simulink model "FYI_Twin_CyberResilient"  (R2025b)
settings: Solver=VariableStepAuto  StartTime=0.0  StopTime=TF  FixedStep=1/120  RelTol=1e-5
PreLoadFcn:
  | [aircraft, state] = astDehavillandBeaver();
  | thrustX = getCoefficient(aircraft,"CX","Propeller",Component="Propeller");
model workspace (MATLAB code in the model file + MAT data in the model file):
  ActuatorCmds = [0.0013469; -0.14185; -0.03733]
  AileronCmd = 0.0013469
  ElevatorCmd = -0.14185
  RudderCmd = -0.03733
  TF = 60
  ThrottleCmd = 0.5
  U0 = 33.0529
  V0 = 0.093272
  W0 = 10.1004
  Xe0 = -2.8165e-12
  Ye0 = 4.3033e-12
  Ze0 = -2202
  aircraft : Aero.FixedWing (value not decoded)
  altitude0 = 2202
  attack_enable = 1
  attack_mode = 3
  blend_rate = 0.05
  inputs0 : object (value not decoded)
  lat0 = 0.843936506509
  lat0_deg = 48.354
  lon0 = 0.205746393542
  lon0_deg = 11.7884
  p0 = 3.0707e-20
  phi0 = 0.0092342
  psi0 = 0
  q0 = 5.1124e-22
  r0 = -8.6217e-20
  required_count = 5
  state : astDehavillandBeaverState (value not decoded)
  states : object (value not decoded)
  states0 : object (value not decoded)
  theta0 = 0.29658
  thrustX : Simulink.LookupTable (value not decoded)
  u_twin = [0.0013469; -0.14185; -0.03733; 0.5; 0.5]
  x0 = [0.0092342; 0.29658; 0; 3.0707e-20; 5.1124e-22; -8.6217e-20; 33.0529; 0.093272; 10.1004; -2.8165e-12; 4.3033e-12; -2202]
  x0_beaver = [0.0092342; 0.29658; 0; 3.0707e-20; 5.1124e-22; -8.6217e-20; 33.0529; 0.093272; 10.1004; -2.8165e-12; 4.3033e-12; -8202]
  x0_unified = [33.0529; 0.093272; 10.1004; 0.0092342; 0.29658; 0; 3.0707e-20; 5.1124e-22; -8.6217e-20; 0.205746393542; 0.843936506509; 2202]
  other statements: initialize6DOFSkyHogg;
symbols that are objects in the model workspace (value not decoded): aircraft, state
undefined symbols (not defined in the file or in its folder): F, Light, MIL
libraries: aerolibasang x6, aerolibobsolete x2, aerolibadyn x2, aerolibatmos2 x2, aerolibwind2 x2, sharedtransform x2, aerolibfltsims x2
(part 2 of 2)

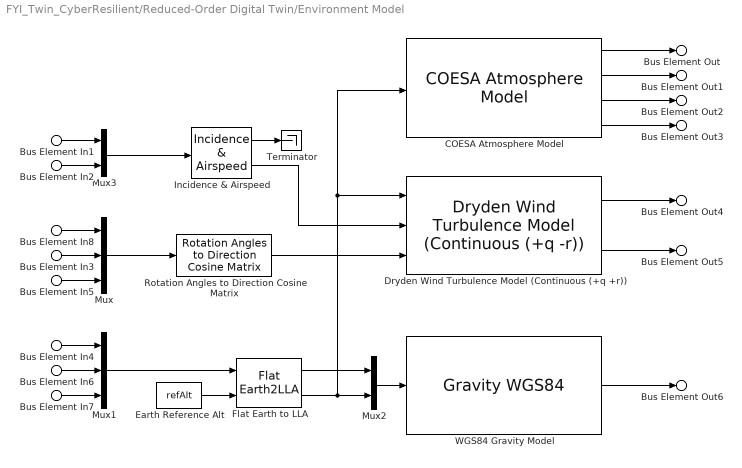
== system FYI_Twin_CyberResilient/Reduced-Order Digital Twin/Environment Model ==
  Bus Element In1 : Inport  PortName=States  Element=u
  Bus Element In2 : Inport  PortName=States  Element=w
  Bus Element In3 : Inport  PortName=States  Element=theta
  Bus Element In4 : Inport  PortName=States  Element=Xe
  Bus Element In7 : Inport  PortName=States  Element=Ze
  Bus Element In8 : Inport  PortName=States  Element=phi
  Bus Element In5 : Inport  PortName=States  Element=psi
  Bus Element In6 : Inport  PortName=States  Element=Ye
  COESA Atmosphere Model : aerolibatmos2/COESA Atmosphere Model  units=Metric (MKS)  spec=1976 COESA-extended U.S. Standard Atmosphere  model=Profile  profile_var=High temperature  profile_percent=1%  profile_alt=5 km (16404 ft)  envelope_var=High temperature  envelope_percent=1%  action=Warning
  Dryden Wind Turbulence Model (Continuous (+q +r)) : aerolibwind2/Dryden Wind Turbulence Model  (Continuous (+q -r))  units=Metric (MKS)  spec=MIL-F-8785C  model=Continuous Dryden (+q -r)  W20=W20  Wdeg=Wdeg  TurbProb=10^-2 - Light  L_high=L_high  Wingspan=Wingspan  ts=ts  Seed=Seed  T_on=off
  Earth Reference Alt : Constant  Value=refAlt
  Flat Earth to LLA : FlatEarth2LLA  R=6378137  LL0=[0 0]
  Incidence & Airspeed : aerolibasang/Incidence  & Airspeed
  Mux : Mux  Inputs=3
  Mux1 : Mux  Inputs=3
  Mux2 : Mux  Inputs=2
  Mux3 : Mux  Inputs=2
  Rotation Angles to Direction Cosine Matrix : sharedtransform/Rotation Angles to Direction Cosine Matrix  rotationOrder=ZYX  aMode=aMode
  Terminator : Terminator
  "WGS84 Gravity Model  " : GravityWGS84
  Bus Element Out : Outport  VectorParamsAs1DForOutWhenUnconnected=off  PortName=Env  Element=To
  Bus Element Out1 : Outport  VectorParamsAs1DForOutWhenUnconnected=off  PortName=Env  Element=a
  Bus Element Out2 : Outport  VectorParamsAs1DForOutWhenUnconnected=off  PortName=Env  Element=Po
  Bus Element Out3 : Outport  VectorParamsAs1DForOutWhenUnconnected=off  PortName=Env  Element=AirDensity
  Bus Element Out4 : Outport  VectorParamsAs1DForOutWhenUnconnected=off  PortName=Env  Element=WindVelocity
  Bus Element Out5 : Outport  VectorParamsAs1DForOutWhenUnconnected=off  PortName=Env  Element=WindAngularRates
  Bus Element Out6 : Outport  VectorParamsAs1DForOutWhenUnconnected=off  PortName=Env  Element=g
  wires:
  Dryden Wind Turbulence Model (Continuous (+q +r))/1 -> Bus Element Out4/1
  Dryden Wind Turbulence Model (Continuous (+q +r))/2 -> Bus Element Out5/1
  Mux2/1 -> "WGS84 Gravity Model  "/1
  Bus Element In4/1 -> Mux1/1
  Bus Element In7/1 -> Mux1/3
  Bus Element In6/1 -> Mux1/2
  Bus Element In5/1 -> Mux/3
  Bus Element In8/1 -> Mux/1
  Bus Element In2/1 -> Mux3/2
  Bus Element In1/1 -> Mux3/1
  "WGS84 Gravity Model  "/1 -> Bus Element Out6/1
  COESA Atmosphere Model/2 -> Bus Element Out1/1
  COESA Atmosphere Model/1 -> Bus Element Out/1
  COESA Atmosphere Model/4 -> Bus Element Out3/1
  COESA Atmosphere Model/3 -> Bus Element Out2/1
  Flat Earth to LLA/1 -> Mux2/1
  Earth Reference Alt/1 -> Flat Earth to LLA/2
  Incidence & Airspeed/2 -> Dryden Wind Turbulence Model (Continuous (+q +r))/2
  Flat Earth to LLA/2 -> Mux2/2, COESA Atmosphere Model/1, Dryden Wind Turbulence Model (Continuous (+q +r))/1
  Mux3/1 -> Incidence & Airspeed/1
  Incidence & Airspeed/1 -> Terminator/1
  Mux/1 -> Rotation Angles to Direction Cosine Matrix/1
  Bus Element In3/1 -> Mux/2
  Rotation Angles to Direction Cosine Matrix/1 -> Dryden Wind Turbulence Model (Continuous (+q +r))/3
  Mux1/1 -> Flat Earth to LLA/1

== system FYI_Twin_CyberResilient/Reduced-Order Digital Twin/Propulsion ==
  cmd : Inport
  Mux : Mux  Inputs=[1 2]
  ThrustX : Lookup_n-D  NumberOfTableDimensions=1  DataSpecification=Lookup table object  LookupTableObject=thrustX  BreakpointsForDimension1="getCoefficient(aircraft,\"CX\",\"Propeller\",Component=\"Propeller\").Breakpoints(1).Value"  IndexSearchMethod=Linear search  BeginIndexSearchUsingPreviousIndexResult=on  Table="getCoefficient(aircraft,\"CX\",\"Propeller\",Component=\"Propeller\").Table.Value"  ExtrapMethod=Clip
  ThrustYZ : Constant  Value=[0 0]'  SampleTime=-1
  Thrust_M1 : Constant  Value=[0 0 0]'  SampleTime=-1
  F : Outport  Unit=N  VectorParamsAs1DForOutWhenUnconnected=off
  M : Outport  Port=2  Unit=N*m  VectorParamsAs1DForOutWhenUnconnected=off
  wires:
  Thrust_M1/1 -> M/1
  ThrustX/1 -> Mux/1
  ThrustYZ/1 -> Mux/2
  Mux/1 -> F/1
  cmd/1 -> ThrustX/1

== system FYI_Twin_CyberResilient/True Aircraft States Adapter/Geodetic Coordinates ==
  VN : Inport
  VE : Inport  Port=2
  VD : Inport  Port=3
  Gain : Gain  Gain=-1
  Integrator : Integrator  InitialCondition=150
  Integrator1 : Integrator  InitialCondition=0.22181
  Integrator2 : Integrator  InitialCondition=1.356068
  LATITUDE : MATLAB Function  TreatAsAtomicUnit=on
  LONGITUDE : MATLAB Function  TreatAsAtomicUnit=on
  M and N : Subsystem
  gamma(Longitude) : Outport
  phi(Latitude) : Outport  Port=2
  h : Outport  Port=3
  wires:
  VD/1 -> Gain/1  "VD"
  Gain/1 -> Integrator/1  "h_dot"
  Integrator/1 -> LATITUDE/3(h), LONGITUDE/3(h), h/1  "h"
  M and N/1(M) -> LATITUDE/2(M)
  M and N/2(N) -> LONGITUDE/2(N)
  LATITUDE/1(phi_dot) -> Integrator1/1  "phi_dot"
  Integrator1/1 -> LONGITUDE/4(phi), M and N/1(phi), phi(Latitude)/1  "phi"
  VE/1 -> LONGITUDE/1(VE)  "VE"
  VN/1 -> LATITUDE/1(VN)  "VN"
  LONGITUDE/1(gamma_dot) -> Integrator2/1  "gamma_dot"
  Integrator2/1 -> gamma(Longitude)/1  "gamma"

== system FYI_Twin_CyberResilient/True Aircraft States Adapter/Navigational BLOCK ==
  U : Inport
  V : Inport  Port=2
  W : Inport  Port=3
  Phi : Inport  Port=4
  Theta : Inport  Port=5
  Psi : Inport  Port=6
  Math Function : Math  Operator=transpose
  Matrix Multiply : Product  Multiplication=Matrix(*)
  Mux2 : Mux  Inputs=3
  Navigational Equation : Subsystem
  V_v : Outport
  wires:
  V/1 -> Mux2/2
  Psi/1 -> Navigational Equation/3(phi)
  W/1 -> Mux2/3
  Navigational Equation/1(C_B/V) -> Math Function/1
  Matrix Multiply/1 -> V_v/1
  Theta/1 -> Navigational Equation/2(theat)
  U/1 -> Mux2/1
  Phi/1 -> Navigational Equation/1(psi)
  Math Function/1 -> Matrix Multiply/1
  Mux2/1 -> Matrix Multiply/2

== system FYI_Twin_CyberResilient/Twin_States_Adapter/Geodetic Coordinates ==
  VN : Inport
  VE : Inport  Port=2
  VD : Inport  Port=3
  Gain : Gain  Gain=-1
  Integrator : Integrator  InitialCondition=150
  Integrator1 : Integrator  InitialCondition=0.22181
  Integrator2 : Integrator  InitialCondition=1.356068
  LATITUDE : MATLAB Function  TreatAsAtomicUnit=on
  LONGITUDE : MATLAB Function  TreatAsAtomicUnit=on
  M and N : Subsystem
  gamma(Longitude) : Outport
  phi(Latitude) : Outport  Port=2
  h : Outport  Port=3
  wires:
  VD/1 -> Gain/1  "VD"
  Gain/1 -> Integrator/1  "h_dot"
  Integrator/1 -> LATITUDE/3(h), LONGITUDE/3(h), h/1  "h"
  M and N/1(M) -> LATITUDE/2(M)
  M and N/2(N) -> LONGITUDE/2(N)
  LATITUDE/1(phi_dot) -> Integrator1/1  "phi_dot"
  Integrator1/1 -> LONGITUDE/4(phi), M and N/1(phi), phi(Latitude)/1  "phi"
  VE/1 -> LONGITUDE/1(VE)  "VE"
  VN/1 -> LATITUDE/1(VN)  "VN"
  LONGITUDE/1(gamma_dot) -> Integrator2/1  "gamma_dot"
  Integrator2/1 -> gamma(Longitude)/1  "gamma"

== system FYI_Twin_CyberResilient/Twin_States_Adapter/Navigational BLOCK ==
  U : Inport
  V : Inport  Port=2
  W : Inport  Port=3
  Phi : Inport  Port=4
  Theta : Inport  Port=5
  Psi : Inport  Port=6
  Math Function : Math  Operator=transpose
  Matrix Multiply : Product  Multiplication=Matrix(*)
  Mux2 : Mux  Inputs=3
  Navigational Equation : Subsystem
  V_v : Outport
  wires:
  V/1 -> Mux2/2
  Psi/1 -> Navigational Equation/3(phi)
  W/1 -> Mux2/3
  Navigational Equation/1(C_B/V) -> Math Function/1
  Matrix Multiply/1 -> V_v/1
  Theta/1 -> Navigational Equation/2(theat)
  U/1 -> Mux2/1
  Phi/1 -> Navigational Equation/1(psi)
  Math Function/1 -> Matrix Multiply/1
  Mux2/1 -> Matrix Multiply/2

== system FYI_Twin_CyberResilient/6-DoF Aircraft Plant/Aerodynamic Model/Actuator Aerodynamic Coefficients ==
  Bus Element In13 : Inport  PortName=ActuatorCmds  Element=Elevator
  Bus Element In1 : Inport  PortName=ActuatorCmds  Element=Aileron
  Bus Element In2 : Inport  PortName=ActuatorCmds  Element=Rudder
  Alpha : Inport  Port=2
  Beta2 : Inport  Port=3
  Aileron : Subsystem
  Constant : Constant  Value=0
  Elevator : Subsystem
  Flap : Subsystem
  Rudder : Subsystem
  Sum : Sum  Inputs=4  InputSameDT=on  SaturateOnIntegerOverflow=on  OutDataTypeStr=Inherit: Same as first input
  Coeff : Outport  InitialOutput=0  VectorParamsAs1DForOutWhenUnconnected=off
  wires:
  Constant/1 -> Flap/1(Actuator)
  Bus Element In2/1 -> Rudder/1(Actuator)
  Bus Element In1/1 -> Aileron/1(Actuator)
  Bus Element In13/1 -> Elevator/1(Actuator)
  Beta2/1 -> Elevator/2(Beta2)
  Flap/1(delCoeff) -> Sum/4
  Alpha/1 -> Flap/2(Alpha), Rudder/2(Alpha), Aileron/2(Alpha)
  Rudder/1(delCoeff) -> Sum/3
  Aileron/1(delCoeff) -> Sum/2
  Elevator/1(delCoeff) -> Sum/1
  Sum/1 -> Coeff/1

== system FYI_Twin_CyberResilient/6-DoF Aircraft Plant/Aerodynamic Model/Aerodynamic Coefficients ==
  Alpha : Inport
  Alpha2 : Inport  Port=2
  Alpha3 : Inport  Port=3
  Beta : Inport  Port=4
  Beta2 : Inport  Port=5
  Beta3 : Inport  Port=6
  V : Inport  Port=7
  pqr : Inport  Port=8  Unit=m/s
  Body Rate Damping : Subsystem
  Datum Coefficients : Subsystem
  Sum : Sum  Inputs=|++
  Coeff : Outport  VectorParamsAs1DForOutWhenUnconnected=off
  wires:
  pqr/1 -> Body Rate Damping/2(pqr)
  Sum/1 -> Coeff/1
  V/1 -> Body Rate Damping/1(V)
  Body Rate Damping/1(Coeff) -> Sum/2
  Datum Coefficients/1(Coeff) -> Sum/1
  Beta/1 -> Datum Coefficients/4(Beta)
  Alpha/1 -> Datum Coefficients/1(Alpha)
  Alpha2/1 -> Datum Coefficients/2(Alpha2)
  Alpha3/1 -> Datum Coefficients/3(Alpha3)
  Beta2/1 -> Datum Coefficients/5(Beta2)
  Beta3/1 -> Datum Coefficients/6(Beta3)

== system FYI_Twin_CyberResilient/6-DoF Aircraft Plant/Aerodynamic Model/Subsystem ==
  Vb : Inport
  "Incidence, Sideslip, & Airspeed" : aerolibasang/Incidence, Sideslip, & Airspeed
  Product{,1..3} (4 alike) : Product
  Alpha : Outport
  Alpha2 : Outport  Port=2
  Alpha3 : Outport  Port=3
  Beta : Outport  Port=4
  Beta2 : Outport  Port=5
  Beta3 : Outport  Port=6
  V : Outport  Port=7
  wires:
  Product/1 -> Product1/1, Alpha2/1
  "Incidence, Sideslip, & Airspeed"/1 -> Product/1, Alpha/1, Product/2, Product1/2
  "Incidence, Sideslip, & Airspeed"/3 -> V/1
  Vb/1 -> "Incidence, Sideslip, & Airspeed"/1
  Product1/1 -> Alpha3/1
  Product2/1 -> Product3/1, Beta2/1
  Product3/1 -> Beta3/1
  "Incidence, Sideslip, & Airspeed"/2 -> Product3/2, Product2/2, Product2/1, Beta/1

== system FYI_Twin_CyberResilient/6-DoF Aircraft Plant/Aerodynamic Model/ToBus ==
  I : Inport
  Bus Creator3 : BusCreator  Inputs=3
  Demux : Demux  Outputs=3
  O : Outport  VectorParamsAs1DForOutWhenUnconnected=off
  wires:
  I/1 -> Demux/1
  Demux/2 -> Bus Creator3/2  "q_wind"
  Bus Creator3/1 -> O/1
  Demux/3 -> Bus Creator3/3  "r_wind"
  Demux/1 -> Bus Creator3/1  "p_wind"

== system FYI_Twin_CyberResilient/Reduced-Order Digital Twin/Aerodynamic Model/Actuator Aerodynamic Coefficients ==
  Bus Element In13 : Inport  PortName=ActuatorCmds  Element=Elevator
  Bus Element In1 : Inport  PortName=ActuatorCmds  Element=Aileron
  Bus Element In2 : Inport  PortName=ActuatorCmds  Element=Rudder
  Alpha : Inport  Port=2
  Beta2 : Inport  Port=3
  Aileron : Subsystem
  Constant : Constant  Value=0
  Elevator : Subsystem
  Flap : Subsystem
  Rudder : Subsystem
  Sum : Sum  Inputs=4  InputSameDT=on  SaturateOnIntegerOverflow=on  OutDataTypeStr=Inherit: Same as first input
  Coeff : Outport  InitialOutput=0  VectorParamsAs1DForOutWhenUnconnected=off
  wires:
  Constant/1 -> Flap/1(Actuator)
  Bus Element In2/1 -> Rudder/1(Actuator)
  Bus Element In1/1 -> Aileron/1(Actuator)
  Bus Element In13/1 -> Elevator/1(Actuator)
  Beta2/1 -> Elevator/2(Beta2)
  Flap/1(delCoeff) -> Sum/4
  Alpha/1 -> Flap/2(Alpha), Rudder/2(Alpha), Aileron/2(Alpha)
  Rudder/1(delCoeff) -> Sum/3
  Aileron/1(delCoeff) -> Sum/2
  Elevator/1(delCoeff) -> Sum/1
  Sum/1 -> Coeff/1

== system FYI_Twin_CyberResilient/Reduced-Order Digital Twin/Aerodynamic Model/Aerodynamic Coefficients ==
  Alpha : Inport
  Alpha2 : Inport  Port=2
  Alpha3 : Inport  Port=3
  Beta : Inport  Port=4
  Beta2 : Inport  Port=5
  Beta3 : Inport  Port=6
  V : Inport  Port=7
  pqr : Inport  Port=8  Unit=m/s
  Body Rate Damping : Subsystem
  Datum Coefficients : Subsystem
  Sum : Sum  Inputs=|++
  Coeff : Outport  VectorParamsAs1DForOutWhenUnconnected=off
  wires:
  pqr/1 -> Body Rate Damping/2(pqr)
  Sum/1 -> Coeff/1
  V/1 -> Body Rate Damping/1(V)
  Body Rate Damping/1(Coeff) -> Sum/2
  Datum Coefficients/1(Coeff) -> Sum/1
  Beta/1 -> Datum Coefficients/4(Beta)
  Alpha/1 -> Datum Coefficients/1(Alpha)
  Alpha2/1 -> Datum Coefficients/2(Alpha2)
  Alpha3/1 -> Datum Coefficients/3(Alpha3)
  Beta2/1 -> Datum Coefficients/5(Beta2)
  Beta3/1 -> Datum Coefficients/6(Beta3)

== system FYI_Twin_CyberResilient/Reduced-Order Digital Twin/Aerodynamic Model/Subsystem ==
  Vb : Inport
  "Incidence, Sideslip, & Airspeed" : aerolibasang/Incidence, Sideslip, & Airspeed
  Product{,1..3} (4 alike) : Product
  Alpha : Outport
  Alpha2 : Outport  Port=2
  Alpha3 : Outport  Port=3
  Beta : Outport  Port=4
  Beta2 : Outport  Port=5
  Beta3 : Outport  Port=6
  V : Outport  Port=7
  wires:
  Product/1 -> Product1/1, Alpha2/1
  "Incidence, Sideslip, & Airspeed"/1 -> Product/1, Alpha/1, Product/2, Product1/2
  "Incidence, Sideslip, & Airspeed"/3 -> V/1
  Vb/1 -> "Incidence, Sideslip, & Airspeed"/1
  Product1/1 -> Alpha3/1
  Product2/1 -> Product3/1, Beta2/1
  Product3/1 -> Beta3/1
  "Incidence, Sideslip, & Airspeed"/2 -> Product3/2, Product2/2, Product2/1, Beta/1

== system FYI_Twin_CyberResilient/Reduced-Order Digital Twin/Aerodynamic Model/ToBus ==
  I : Inport
  Bus Creator3 : BusCreator  Inputs=3
  Demux : Demux  Outputs=3
  O : Outport  VectorParamsAs1DForOutWhenUnconnected=off
  wires:
  I/1 -> Demux/1
  Demux/2 -> Bus Creator3/2  "q_wind"
  Bus Creator3/1 -> O/1
  Demux/3 -> Bus Creator3/3  "r_wind"
  Demux/1 -> Bus Creator3/1  "p_wind"

== system FYI_Twin_CyberResilient/True Aircraft States Adapter/Geodetic Coordinates/M and N ==
  phi : Inport
  Constant : Constant  Value=0.081819190842622
  M and N : MATLAB Function  TreatAsAtomicUnit=on
  a : Constant  Value=6378137
  M : Outport
  N : Outport  Port=2
  wires:
  Constant/1 -> M and N/2(e)
  phi/1 -> M and N/3(phi)
  M and N/1(M) -> M/1
  a/1 -> M and N/1(a)
  M and N/2(N) -> N/1

== system FYI_Twin_CyberResilient/True Aircraft States Adapter/Navigational BLOCK/Navigational Equation ==
  psi : Inport
  theat : Inport  Port=2
  phi : Inport  Port=3
  Matrix Multiply : Product  Inputs=3  Multiplication=Matrix(*)
  Roationa Matrix from 2 to body : MATLAB Function  TreatAsAtomicUnit=on
  Roational Matrix from 1 to 2 : MATLAB Function  TreatAsAtomicUnit=on
  Rotaional Matrix from V to 1 : MATLAB Function  TreatAsAtomicUnit=on
  C_B/V : Outport
  wires:
  psi/1 -> Rotaional Matrix from V to 1/1(psi)
  theat/1 -> Roational Matrix from 1 to 2/1(theta)
  phi/1 -> Roationa Matrix from 2 to body/1(phi)
  Roationa Matrix from 2 to body/1(C_b_2) -> Matrix Multiply/1
  Roational Matrix from 1 to 2/1(C_2_1) -> Matrix Multiply/2
  Rotaional Matrix from V to 1/1(C_1_V) -> Matrix Multiply/3
  Matrix Multiply/1 -> C_B/V/1

== system FYI_Twin_CyberResilient/Twin_States_Adapter/Geodetic Coordinates/M and N ==
  phi : Inport
  Constant : Constant  Value=0.081819190842622
  M and N : MATLAB Function  TreatAsAtomicUnit=on
  a : Constant  Value=6378137
  M : Outport
  N : Outport  Port=2
  wires:
  Constant/1 -> M and N/2(e)
  phi/1 -> M and N/3(phi)
  M and N/1(M) -> M/1
  a/1 -> M and N/1(a)
  M and N/2(N) -> N/1

== system FYI_Twin_CyberResilient/Twin_States_Adapter/Navigational BLOCK/Navigational Equation ==
  psi : Inport
  theat : Inport  Port=2
  phi : Inport  Port=3
  Matrix Multiply : Product  Inputs=3  Multiplication=Matrix(*)
  Roationa Matrix from 2 to body : MATLAB Function  TreatAsAtomicUnit=on
  Roational Matrix from 1 to 2 : MATLAB Function  TreatAsAtomicUnit=on
  Rotaional Matrix from V to 1 : MATLAB Function  TreatAsAtomicUnit=on
  C_B/V : Outport
  wires:
  psi/1 -> Rotaional Matrix from V to 1/1(psi)
  theat/1 -> Roational Matrix from 1 to 2/1(theta)
  phi/1 -> Roationa Matrix from 2 to body/1(phi)
  Roationa Matrix from 2 to body/1(C_b_2) -> Matrix Multiply/1
  Roational Matrix from 1 to 2/1(C_2_1) -> Matrix Multiply/2
  Rotaional Matrix from V to 1/1(C_1_V) -> Matrix Multiply/3
  Matrix Multiply/1 -> C_B/V/1

== system FYI_Twin_CyberResilient/6-DoF Aircraft Plant/Aerodynamic Model/Actuator Aerodynamic Coefficients/Aileron ==
  Actuator : Inport
  Alpha : Inport  Port=2
  Constant : Constant  Value=aircraft.Surfaces(1).Surfaces(1).Coefficients.Table.Variables
  Matrix Multiply : Product  Multiplication=Matrix(*)
  Product : Product
  Vector Concatenate : Concatenate
  delCoeff : Outport  VectorParamsAs1DForOutWhenUnconnected=off
  wires:
  Actuator/1 -> Product/1, Vector Concatenate/1
  Alpha/1 -> Product/2
  Vector Concatenate/1 -> Matrix Multiply/2
  Matrix Multiply/1 -> delCoeff/1
  Product/1 -> Vector Concatenate/2
  Constant/1 -> Matrix Multiply/1

== system FYI_Twin_CyberResilient/6-DoF Aircraft Plant/Aerodynamic Model/Actuator Aerodynamic Coefficients/Elevator ==
  Actuator : Inport
  Beta2 : Inport  Port=2
  Constant : Constant  Value=aircraft.Surfaces(2).Surfaces(1).Coefficients.Table.Variables
  Matrix Multiply : Product  Multiplication=Matrix(*)
  Product : Product
  Vector Concatenate : Concatenate
  delCoeff : Outport  VectorParamsAs1DForOutWhenUnconnected=off
  wires:
  Matrix Multiply/1 -> delCoeff/1
  Constant/1 -> Matrix Multiply/1
  Vector Concatenate/1 -> Matrix Multiply/2
  Actuator/1 -> Product/1, Vector Concatenate/1
  Beta2/1 -> Product/2
  Product/1 -> Vector Concatenate/2

== system FYI_Twin_CyberResilient/6-DoF Aircraft Plant/Aerodynamic Model/Actuator Aerodynamic Coefficients/Flap ==
  Actuator : Inport
  Alpha : Inport  Port=2
  Constant : Constant  Value=aircraft.Surfaces(1).Surfaces(2).Coefficients.Table.Variables
  Matrix Multiply : Product  Multiplication=Matrix(*)
  Product : Product
  Vector Concatenate : Concatenate
  delCoeff : Outport  VectorParamsAs1DForOutWhenUnconnected=off
  wires:
  Actuator/1 -> Product/1, Vector Concatenate/1
  Alpha/1 -> Product/2
  Vector Concatenate/1 -> Matrix Multiply/2
  Matrix Multiply/1 -> delCoeff/1
  Product/1 -> Vector Concatenate/2
  Constant/1 -> Matrix Multiply/1

== system FYI_Twin_CyberResilient/6-DoF Aircraft Plant/Aerodynamic Model/Actuator Aerodynamic Coefficients/Rudder ==
  Actuator : Inport
  Alpha : Inport  Port=2
  Constant : Constant  Value=aircraft.Surfaces(3).Surfaces(1).Coefficients.Table.Variables
  Matrix Multiply : Product  Multiplication=Matrix(*)
  Product : Product
  Vector Concatenate : Concatenate
  delCoeff : Outport  VectorParamsAs1DForOutWhenUnconnected=off
  wires:
  Actuator/1 -> Product/1, Vector Concatenate/1
  Alpha/1 -> Product/2
  Vector Concatenate/1 -> Matrix Multiply/2
  Matrix Multiply/1 -> delCoeff/1
  Product/1 -> Vector Concatenate/2
  Constant/1 -> Matrix Multiply/1

== system FYI_Twin_CyberResilient/6-DoF Aircraft Plant/Aerodynamic Model/Aerodynamic Coefficients/Body Rate Damping ==
  V : Inport  Unit=m/s
  Bus Element In : Inport  Port=2  PortName=pqr  Element=p_wind
  Bus Element In1 : Inport  Port=2  PortName=pqr  Element=q_wind
  Bus Element In2 : Inport  Port=2  PortName=pqr  Element=r_wind
  Constant : Constant  Value="aircraft.Coefficients.Table{:, [\"pb2V\", \"qcV\", \"rb2V\"]}"
  Matrix Multiply : Product  Multiplication=Matrix(*)
  Product1 : Product
  Product2 : Product
  Product3 : Product
  Subsystem : Subsystem
  Vector Concatenate : Concatenate  NumInputs=3
  Coeff : Outport  InitialOutput=0  VectorParamsAs1DForOutWhenUnconnected=off
  wires:
  Matrix Multiply/1 -> Coeff/1
  Vector Concatenate/1 -> Matrix Multiply/2
  Product1/1 -> Vector Concatenate/1  "pb2V"
  Bus Element In/1 -> Product1/1
  Product2/1 -> Vector Concatenate/2  "qcV"
  Subsystem/2(b2V) -> Product3/2, Product1/2
  Product3/1 -> Vector Concatenate/3  "rb2V"
  Constant/1 -> Matrix Multiply/1
  Bus Element In1/1 -> Product2/1
  Subsystem/1(cV) -> Product2/2
  Bus Element In2/1 -> Product3/1
  V/1 -> Subsystem/1(V)

== system FYI_Twin_CyberResilient/6-DoF Aircraft Plant/Aerodynamic Model/Aerodynamic Coefficients/Datum Coefficients ==
  Alpha : Inport
  Alpha2 : Inport  Port=2
  Alpha3 : Inport  Port=3
  Beta : Inport  Port=4
  Beta2 : Inport  Port=5
  Beta3 : Inport  Port=6
  Constant : Constant  Value=aircraft.Coefficients.Table.Zero
  Constant2 : Constant  Value="aircraft.Coefficients.Table{:,[\"Alpha\",\"Alpha2\",\"Alpha3\",\"Beta\",\"Beta2\",\"Beta3\"]}"
  Matrix Multiply : Product  Multiplication=Matrix(*)
  Sum : Sum  Inputs=++|
  Vector Concatenate : Concatenate  NumInputs=6
  Coeff : Outport  InitialOutput=0  VectorParamsAs1DForOutWhenUnconnected=off
  wires:
  Sum/1 -> Coeff/1
  Constant/1 -> Sum/1
  Matrix Multiply/1 -> Sum/2
  Alpha/1 -> Vector Concatenate/1
  Vector Concatenate/1 -> Matrix Multiply/2
  Constant2/1 -> Matrix Multiply/1
  Beta/1 -> Vector Concatenate/4
  Alpha3/1 -> Vector Concatenate/3
  Alpha2/1 -> Vector Concatenate/2
  Beta2/1 -> Vector Concatenate/5
  Beta3/1 -> Vector Concatenate/6

== system FYI_Twin_CyberResilient/Reduced-Order Digital Twin/Aerodynamic Model/Actuator Aerodynamic Coefficients/Aileron ==
  Actuator : Inport
  Alpha : Inport  Port=2
  Constant : Constant  Value=aircraft.Surfaces(1).Surfaces(1).Coefficients.Table.Variables
  Matrix Multiply : Product  Multiplication=Matrix(*)
  Product : Product
  Vector Concatenate : Concatenate
  delCoeff : Outport  VectorParamsAs1DForOutWhenUnconnected=off
  wires:
  Actuator/1 -> Product/1, Vector Concatenate/1
  Alpha/1 -> Product/2
  Vector Concatenate/1 -> Matrix Multiply/2
  Matrix Multiply/1 -> delCoeff/1
  Product/1 -> Vector Concatenate/2
  Constant/1 -> Matrix Multiply/1

== system FYI_Twin_CyberResilient/Reduced-Order Digital Twin/Aerodynamic Model/Actuator Aerodynamic Coefficients/Elevator ==
  Actuator : Inport
  Beta2 : Inport  Port=2
  Constant : Constant  Value=aircraft.Surfaces(2).Surfaces(1).Coefficients.Table.Variables
  Matrix Multiply : Product  Multiplication=Matrix(*)
  Product : Product
  Vector Concatenate : Concatenate
  delCoeff : Outport  VectorParamsAs1DForOutWhenUnconnected=off
  wires:
  Matrix Multiply/1 -> delCoeff/1
  Constant/1 -> Matrix Multiply/1
  Vector Concatenate/1 -> Matrix Multiply/2
  Actuator/1 -> Product/1, Vector Concatenate/1
  Beta2/1 -> Product/2
  Product/1 -> Vector Concatenate/2

== system FYI_Twin_CyberResilient/Reduced-Order Digital Twin/Aerodynamic Model/Actuator Aerodynamic Coefficients/Flap ==
  Actuator : Inport
  Alpha : Inport  Port=2
  Constant : Constant  Value=aircraft.Surfaces(1).Surfaces(2).Coefficients.Table.Variables
  Matrix Multiply : Product  Multiplication=Matrix(*)
  Product : Product
  Vector Concatenate : Concatenate
  delCoeff : Outport  VectorParamsAs1DForOutWhenUnconnected=off
  wires:
  Actuator/1 -> Product/1, Vector Concatenate/1
  Alpha/1 -> Product/2
  Vector Concatenate/1 -> Matrix Multiply/2
  Matrix Multiply/1 -> delCoeff/1
  Product/1 -> Vector Concatenate/2
  Constant/1 -> Matrix Multiply/1

== system FYI_Twin_CyberResilient/Reduced-Order Digital Twin/Aerodynamic Model/Actuator Aerodynamic Coefficients/Rudder ==
  Actuator : Inport
  Alpha : Inport  Port=2
  Constant : Constant  Value=aircraft.Surfaces(3).Surfaces(1).Coefficients.Table.Variables
  Matrix Multiply : Product  Multiplication=Matrix(*)
  Product : Product
  Vector Concatenate : Concatenate
  delCoeff : Outport  VectorParamsAs1DForOutWhenUnconnected=off
  wires:
  Actuator/1 -> Product/1, Vector Concatenate/1
  Alpha/1 -> Product/2
  Vector Concatenate/1 -> Matrix Multiply/2
  Matrix Multiply/1 -> delCoeff/1
  Product/1 -> Vector Concatenate/2
  Constant/1 -> Matrix Multiply/1

== system FYI_Twin_CyberResilient/Reduced-Order Digital Twin/Aerodynamic Model/Aerodynamic Coefficients/Body Rate Damping ==
  V : Inport  Unit=m/s
  Bus Element In : Inport  Port=2  PortName=pqr  Element=p_wind
  Bus Element In1 : Inport  Port=2  PortName=pqr  Element=q_wind
  Bus Element In2 : Inport  Port=2  PortName=pqr  Element=r_wind
  Constant : Constant  Value="aircraft.Coefficients.Table{:, [\"pb2V\", \"qcV\", \"rb2V\"]}"
  Matrix Multiply : Product  Multiplication=Matrix(*)
  Product1 : Product
  Product2 : Product
  Product3 : Product
  Subsystem : Subsystem
  Vector Concatenate : Concatenate  NumInputs=3
  Coeff : Outport  InitialOutput=0  VectorParamsAs1DForOutWhenUnconnected=off
  wires:
  Matrix Multiply/1 -> Coeff/1
  Vector Concatenate/1 -> Matrix Multiply/2
  Product1/1 -> Vector Concatenate/1  "pb2V"
  Bus Element In/1 -> Product1/1
  Product2/1 -> Vector Concatenate/2  "qcV"
  Subsystem/2(b2V) -> Product3/2, Product1/2
  Product3/1 -> Vector Concatenate/3  "rb2V"
  Constant/1 -> Matrix Multiply/1
  Bus Element In1/1 -> Product2/1
  Subsystem/1(cV) -> Product2/2
  Bus Element In2/1 -> Product3/1
  V/1 -> Subsystem/1(V)

== system FYI_Twin_CyberResilient/Reduced-Order Digital Twin/Aerodynamic Model/Aerodynamic Coefficients/Datum Coefficients ==
  Alpha : Inport
  Alpha2 : Inport  Port=2
  Alpha3 : Inport  Port=3
  Beta : Inport  Port=4
  Beta2 : Inport  Port=5
  Beta3 : Inport  Port=6
  Constant : Constant  Value=aircraft.Coefficients.Table.Zero
  Constant2 : Constant  Value="aircraft.Coefficients.Table{:,[\"Alpha\",\"Alpha2\",\"Alpha3\",\"Beta\",\"Beta2\",\"Beta3\"]}"
  Matrix Multiply : Product  Multiplication=Matrix(*)
  Sum : Sum  Inputs=++|
  Vector Concatenate : Concatenate  NumInputs=6
  Coeff : Outport  InitialOutput=0  VectorParamsAs1DForOutWhenUnconnected=off
  wires:
  Sum/1 -> Coeff/1
  Constant/1 -> Sum/1
  Matrix Multiply/1 -> Sum/2
  Alpha/1 -> Vector Concatenate/1
  Vector Concatenate/1 -> Matrix Multiply/2
  Constant2/1 -> Matrix Multiply/1
  Beta/1 -> Vector Concatenate/4
  Alpha3/1 -> Vector Concatenate/3
  Alpha2/1 -> Vector Concatenate/2
  Beta2/1 -> Vector Concatenate/5
  Beta3/1 -> Vector Concatenate/6

== system FYI_Twin_CyberResilient/6-DoF Aircraft Plant/Aerodynamic Model/Aerodynamic Coefficients/Body Rate Damping/Subsystem ==
  V : Inport
  Constant1 : Constant  Value=aircraft.ReferenceSpan
  Constant2 : Constant  Value=aircraft.ReferenceLength
  Divide : Product  Inputs=*/
  Gain1 : Gain  Gain=1/2
  Product : Product  Inputs=*/
  cV : Outport
  b2V : Outport  Port=2
  wires:
  Product/1 -> cV/1
  Constant1/1 -> Gain1/1
  V/1 -> Divide/2, Product/2
  Divide/1 -> b2V/1
  Constant2/1 -> Product/1
  Gain1/1 -> Divide/1

== system FYI_Twin_CyberResilient/Reduced-Order Digital Twin/Aerodynamic Model/Aerodynamic Coefficients/Body Rate Damping/Subsystem ==
  V : Inport
  Constant1 : Constant  Value=aircraft.ReferenceSpan
  Constant2 : Constant  Value=aircraft.ReferenceLength
  Divide : Product  Inputs=*/
  Gain1 : Gain  Gain=1/2
  Product : Product  Inputs=*/
  cV : Outport
  b2V : Outport  Port=2
  wires:
  Product/1 -> cV/1
  Constant1/1 -> Gain1/1
  V/1 -> Divide/2, Product/2
  Divide/1 -> b2V/1
  Constant2/1 -> Product/1
  Gain1/1 -> Divide/1

== matlab function FYI_Twin_CyberResilient/Twin_States_Adapter/Geodetic Coordinates/M and N/M and N ==
  data: a input; M output; e input; phi input; N output
function[M,N]=M_N(a,e,phi)

M=(a*(1-e*2)/(1-(e^2)*sin(phi))^3/2);  % Meridian Radius of Curvature

N=a/(1-(e^2)*(sin(phi)^2))^3/2;        % Prime verical radius of curvature

end

== matlab function FYI_Twin_CyberResilient/Twin_States_Adapter/Navigational BLOCK/Navigational Equation/Roationa Matrix from 2 to body ==
  data: phi input; C_b_2 output
function C_b_2 = fcn(phi)

% Roational Matrix from the 2 frame to body frame
C_b_2=[1 0 0; 0 cos(phi) sin(phi); 0 -sin(phi) cos(phi)];
end

== matlab function FYI_Twin_CyberResilient/Twin_States_Adapter/Navigational BLOCK/Navigational Equation/Roational Matrix from 1 to 2 ==
  data: theta input; C_2_1 output
function C_2_1 = fcn(theta)

% Roational Matrix From the 1 frame to 2 frame

C_2_1=[cos(theta) 0 -sin(theta); 0 1 0; sin(theta) 0 cos(theta)];

end

== matlab function FYI_Twin_CyberResilient/Twin_States_Adapter/Navigational BLOCK/Navigational Equation/Rotaional Matrix from V to 1 ==
  data: psi input; C_1_V output
function C_1_V = fcn(psi)

% Calculating the Rotaional Matrix  from the NED to 1 frame

C_1_V=[cos(psi) sin(psi) 0; -sin(psi) cos(psi) 0; 0 0 1];

end

== matlab function FYI_Twin_CyberResilient/Cyber Attack Injection/MATLAB Function ==
  data: x_meas_clean input; x_meas_attacked output; attack_enable input; attack_mode input; t input
function x_meas_attacked = AttackInjectionFcn(x_meas_clean, attack_enable, attack_mode, t)
%--------------------------------------------------------------------------
% Attack modes:
% 0 = no attack
% 1 = altitude spoof
% 2 = air-data spoof
% 3 = coordinated false climb
%--------------------------------------------------------------------------

x = x_meas_clean(:);

x_meas_attacked = zeros(12,1);
x_meas_attacked(:) = x;

attack_start_time = 14.0;

if attack_enable == 1 && t >= attack_start_time

    if attack_mode == 1
        % Altitude spoof only
        x_meas_attacked(12) = x_meas_attacked(12) + 100.0;

    elseif attack_mode == 2
        % Air-data spoof
        x_meas_attacked(1) = x_meas_attacked(1) + 8.0;
        x_meas_attacked(3) = x_meas_attacked(3) - 3.0;

    elseif attack_mode == 3
        % Coordinated false climb
        x_meas_attacked(1)  = x_meas_attacked(1)  + 8.0;
        x_meas_attacked(3)  = x_meas_attacked(3)  - 3.0;
        x_meas_attacked(5)  = x_meas_attacked(5)  + 5*pi/180;
        x_meas_attacked(12) = x_meas_attacked(12) + 50.0;
    end
end

end

== matlab function FYI_Twin_CyberResilient/True Aircraft States Adapter/Navigational BLOCK/Navigational Equation/Roational Matrix from 1 to 2 ==
  data: theta input; C_2_1 output
function C_2_1 = fcn(theta)

% Roational Matrix From the 1 frame to 2 frame

C_2_1=[cos(theta) 0 -sin(theta); 0 1 0; sin(theta) 0 cos(theta)];

end

== matlab function FYI_Twin_CyberResilient/Resilient Autonomy Mode/RAMLogic ==
  data: cyber_flag input; ram_blend input; RAM_active output size=[1 1]; x_meas_attacked input; x_pred_unified input; x_safe output
function [RAM_active, x_safe] = RAMLogicFcn(cyber_flag, ram_blend, x_meas_attacked, x_pred_unified)
%--------------------------------------------------------------------------
% Resilient Autonomy Mode without persistent variables
%
% cyber_flag = 0:
%   x_safe = measured/possibly attacked state
%
% cyber_flag = 1:
%   x_safe transitions smoothly toward twin-predicted trusted state
%   using externally generated ram_blend.
%
% Inputs:
% cyber_flag       : scalar
% ram_blend        : scalar, 0 to 1
% x_meas_attacked  : [12x1]
% x_pred_unified   : [12x1]
%
% Outputs:
% RAM_active       : scalar
% x_safe           : [12x1]
%--------------------------------------------------------------------------

RAM_active = 0.0;
x_safe = zeros(12,1);

if cyber_flag >= 0.5
    RAM_active = 1.0;
else
    RAM_active = 0.0;
end

% Limit blend for safety
if ram_blend < 0.0
    ram_blend = 0.0;
elseif ram_blend > 1.0
    ram_blend = 1.0;
end

for i = 1:12
    x_safe(i) = (1.0 - ram_blend) * x_meas_attacked(i) + ...
                 ram_blend  * x_pred_unified(i);
end

end

== matlab function FYI_Twin_CyberResilient/RAM Command Manager/MATLAB Function ==
  data: RAM_active input; aileron_out output; aileron_in input; elevator_in input; rudder_in input; throttle_in input; elevator_out output; rudder_out output; throttle_out output
function [aileron_out, elevator_out, rudder_out, throttle_out] = RAMCommandManagerFcn(RAM_active, aileron_in, elevator_in, rudder_in, throttle_in)
%--------------------------------------------------------------------------
% RAMCommandManagerFcn
%
% Simple envelope-protected fallback command manager.
% In normal mode, passes commands through.
% In RAM mode, limits command magnitude and keeps trim-biased safe flight.
%--------------------------------------------------------------------------

% Trim/fallback values
aileron_trim  = 0.0013469;
elevator_trim = -0.14185;
rudder_trim   = -0.03733;
throttle_trim = 0.5;

if RAM_active >= 0.5

    % In RAM: revert toward stable trimmed commands
    aileron_out  = aileron_trim;
    elevator_out = elevator_trim;
    rudder_out   = rudder_trim;
    throttle_out = throttle_trim;

else

    % Normal operation
    aileron_out  = aileron_in;
    elevator_out = elevator_in;
    rudder_out   = rudder_in;
    throttle_out = throttle_in;

end

end

== matlab function FYI_Twin_CyberResilient/Reduced-Order Digital Twin/Reduced_Twin_Propulsion ==
  data: cmd input; F output; M output
function [F, M] = ReducedPropulsionFcn(cmd)
% Reduced propulsion model for the digital twin.
% Single-axis thrust only, no engine moment.

F = zeros(3,1);
M = zeros(3,1);

Tmax = 4603;       % N, tune between 3500 and 7000 if needed

throttle = cmd;

if throttle < 0
    throttle = 0;
elseif throttle > 1
    throttle = 1;
end

F(1) = Tmax * throttle;
F(2) = 0;
F(3) = 0;

M(1) = 0;
M(2) = 0;
M(3) = 0;

end

== matlab function FYI_Twin_CyberResilient/Post_RAM_Consistency_Monitor/MATLAB Function ==
  data: x_safe input size=[12 1]; post_RAM_residual_selected output size=[8 1]; x_pred_unified input size=[12 1]; post_RAM_residual_norm output size=[1 1]
function [post_RAM_residual_selected, post_RAM_residual_norm] = PostRAMResidualFcn(x_safe, x_pred_unified)
%--------------------------------------------------------------------------
% PostRAMResidualFcn
%
% Computes residual after RAM trusted-state selection.
%
% State order:
% x = [u; v; w; phi; theta; psi; p; q; r; lon; lat; h]
%
% residual order:
% 1 u
% 2 w
% 3 theta
% 4 q
% 5 altitude
% 6 phi
% 7 p
% 8 r
%--------------------------------------------------------------------------

post_RAM_residual_selected = zeros(8,1);
post_RAM_residual_norm = 0.0;

post_RAM_residual_selected(1) = abs(x_safe(1)  - x_pred_unified(1));    % u
post_RAM_residual_selected(2) = abs(x_safe(3)  - x_pred_unified(3));    % w
post_RAM_residual_selected(3) = abs(x_safe(5)  - x_pred_unified(5));    % theta
post_RAM_residual_selected(4) = abs(x_safe(8)  - x_pred_unified(8));    % q
post_RAM_residual_selected(5) = abs(x_safe(12) - x_pred_unified(12));   % altitude
post_RAM_residual_selected(6) = abs(x_safe(4)  - x_pred_unified(4));    % phi
post_RAM_residual_selected(7) = abs(x_safe(7)  - x_pred_unified(7));    % p
post_RAM_residual_selected(8) = abs(x_safe(9)  - x_pred_unified(9));    % r

for i = 1:8
    post_RAM_residual_norm = post_RAM_residual_norm + post_RAM_residual_selected(i)^2;
end

post_RAM_residual_norm = sqrt(post_RAM_residual_norm);

end

== matlab function FYI_Twin_CyberResilient/Twin_States_Adapter/SensorModelFcn ==
  data: x_true_unified input size=[12 1]; x_pred output size=[12 1]; t input size=[1 1]
function x_pred = SensorModelFcn(x_true_unified, t)
%--------------------------------------------------------------------------
% SensorModelFcn
%
% Adds small deterministic sensor imperfections to true aircraft states.
%
% State order:
% x = [u; v; w; phi; theta; psi; p; q; r; lon; lat; h]
%--------------------------------------------------------------------------

%% Fixed output size
x_pred = zeros(12,1);

%% Extract states

u     = x_true_unified(1);
v     = x_true_unified(2);
w     = x_true_unified(3);

phi   = x_true_unified(4);
theta = x_true_unified(5);
psi   = x_true_unified(6);

p     = x_true_unified(7);
q     = x_true_unified(8);
r     = x_true_unified(9);

lon   = x_true_unified(10);
lat   = x_true_unified(11);
h     = x_true_unified(12);

%% Fixed sensor biases

u_bias = 0.08;        % m/s
v_bias = 0.02;        % m/s
w_bias = 0.03;        % m/s

phi_bias   = deg2rad(0.02);
theta_bias = deg2rad(-20);
psi_bias   = deg2rad(0.05);

p_bias = 0.00015;     % rad/s
q_bias = 0.00015;     % rad/s
r_bias = 0.00015;     % rad/s

lon_bias = deg2rad(0.000001);
lat_bias = deg2rad(0.000001);
h_bias   = 0.40;      % m

%% Small deterministic sensor noise/ripple

u_noise     = 0; %0.04 * 8*sin(0.7*t);
v_noise     = 0; %0.02 * sin(0.5*t);
w_noise     = 0.03 %* sin(0.6*t);

phi_noise   = 0; %deg2rad(0.01)  * sin(0.8*t);
theta_noise = 0; %deg2rad(0.015) * sin(0.9*t);
psi_noise   = 0; %deg2rad(0.02)  * sin(0.4*t);

p_noise = 0.00005 %*sin(0.6*t);
q_noise = 0.00005 %* sin(0.9*t);
r_noise = 0.00005 %*sin(0.7*t);

lon_noise = deg2rad(0.0000003) * sin(0.3*t);
lat_noise = deg2rad(0.0000003) * sin(0.35*t);
h_noise   = 0.25 * sin(0.2*t);

%% Output measured state

x_pred(1)  = u     + u_bias     + u_noise;
x_pred(2)  = v     + v_bias     + v_noise;
x_pred(3)  = w     + w_bias     + w_noise;

x_pred(4)  = phi   + phi_bias   + phi_noise;
x_pred(5)  = theta + theta_bias + theta_noise;
x_pred(6)  = psi   + psi_bias   + psi_noise;

x_pred(7)  = p     + p_bias     + p_noise;
x_pred(8)  = q     + q_bias     + q_noise;
x_pred(9)  = r     + r_bias     + r_noise;

x_pred(10) = lon   + lon_bias   + lon_noise;
x_pred(11) = lat   + lat_bias   + lat_noise;
x_pred(12) = h     + h_bias     + h_noise;

end

== matlab function FYI_Twin_CyberResilient/True Aircraft States Adapter/Navigational BLOCK/Navigational Equation/Rotaional Matrix from V to 1 ==
  data: psi input; C_1_V output
function C_1_V = fcn(psi)

% Calculating the Rotaional Matrix  from the NED to 1 frame

C_1_V=[cos(psi) sin(psi) 0; -sin(psi) cos(psi) 0; 0 0 1];

end

== matlab function FYI_Twin_CyberResilient/True Aircraft States Adapter/Navigational BLOCK/Navigational Equation/Roationa Matrix from 2 to body ==
  data: phi input; C_b_2 output
function C_b_2 = fcn(phi)

% Roational Matrix from the 2 frame to body frame
C_b_2=[1 0 0; 0 cos(phi) sin(phi); 0 -sin(phi) cos(phi)];
end

== matlab function FYI_Twin_CyberResilient/True Aircraft States Adapter/Geodetic Coordinates/M and N/M and N ==
  data: a input; M output; e input; phi input; N output
function[M,N]=M_N(a,e,phi)

M=(a*(1-e*2)/(1-(e^2)*sin(phi))^3/2);  % Meridian Radius of Curvature

N=a/(1-(e^2)*(sin(phi)^2))^3/2;        % Prime verical radius of curvature

end

== matlab function FYI_Twin_CyberResilient/True Aircraft States Adapter/Geodetic Coordinates/LATITUDE ==
  data: VN input; phi_dot output; M input; h input
function phi_dot =Latitude_Rate(VN,M,h)
% Calculating the Rate of change of Latitude

phi_dot=VN/(M+h);
end

== matlab function FYI_Twin_CyberResilient/True Aircraft States Adapter/Geodetic Coordinates/LONGITUDE ==
  data: VE input; gamma_dot output; N input; h input; phi input
function gamma_dot =Longitude_Rate(VE,N,h,phi)

% Calculating the Rate of change of the Longitude

gamma_dot=VE/((N+h)*cos(phi));
end

== matlab function FYI_Twin_CyberResilient/Sensor Model/SensorModelFcn ==
  data: x_true input size=[12 1]; x_meas output size=[12 1]; t input size=[1 1]
function x_meas = SensorModelFcn(x_true, t)
%--------------------------------------------------------------------------
% SensorModelFcn
%
% Adds small deterministic sensor imperfections to true aircraft states.
%
% State order:
% x = [u; v; w; phi; theta; psi; p; q; r; lon; lat; h]
%--------------------------------------------------------------------------

%% Fixed output size
x_meas = zeros(12,1);

%% Extract states

u     = x_true(1);
v     = x_true(2);
w     = x_true(3);

phi   = x_true(4);
theta = x_true(5);
psi   = x_true(6);

p     = x_true(7);
q     = x_true(8);
r     = x_true(9);

lon   = x_true(10);
lat   = x_true(11);
h     = x_true(12);

%% Fixed sensor biases

u_bias = 0.08;        % m/s
v_bias = 0.02;        % m/s
w_bias = 0.03;        % m/s

phi_bias   = deg2rad(0.02);
theta_bias = deg2rad(-20);
psi_bias   = deg2rad(0.05);

p_bias = 0.00015;     % rad/s
q_bias = 0.00015;     % rad/s
r_bias = 0.00015;     % rad/s

lon_bias = deg2rad(0.000001);
lat_bias = deg2rad(0.000001);
h_bias   = 0.40;      % m

%% Small deterministic sensor noise/ripple

u_noise     = 0.04 * 8*sin(0.7*t);
v_noise     = 0.02 * sin(0.5*t);
w_noise     = 0.03 * sin(0.6*t);

phi_noise   = deg2rad(0.01)  * sin(0.8*t);
theta_noise = deg2rad(0.015) * sin(0.9*t);
psi_noise   = deg2rad(0.02)  * sin(0.4*t);

p_noise = 0.00005 * 6*sin(0.6*t);
q_noise = 0.00005 * sin(0.9*t);
r_noise = 0.00005 * 9*sin(0.7*t);

lon_noise = deg2rad(0.0000003) * sin(0.3*t);
lat_noise = deg2rad(0.0000003) * sin(0.35*t);
h_noise   = 0.25 * sin(0.2*t);

%% Output measured state

x_meas(1)  = u     + u_bias     + u_noise;
x_meas(2)  = v     + v_bias     + v_noise;
x_meas(3)  = w     + w_bias     + w_noise;

x_meas(4)  = phi   + phi_bias   + phi_noise;
x_meas(5)  = theta + theta_bias + theta_noise;
x_meas(6)  = psi   + psi_bias   + psi_noise;

x_meas(7)  = p     + p_bias     + p_noise;
x_meas(8)  = q     + q_bias     + q_noise;
x_meas(9)  = r     + r_bias     + r_noise;

x_meas(10) = lon   + lon_bias   + lon_noise;
x_meas(11) = lat   + lat_bias   + lat_noise;
x_meas(12) = h     + h_bias     + h_noise;

end

== matlab function FYI_Twin_CyberResilient/Physics Consistency Monitor/ResidualMonitorFcn ==
  data: x_meas_attacked input; residual_selected output size=8; x_pred_unified input; residual_norm output; exceeded_raw output size=[1 1]
function [residual_selected, residual_norm, exceeded_raw] = ResidualMonitorFcn(x_meas_attacked, x_pred_unified)
%--------------------------------------------------------------------------
% Physics Consistency Monitor
%
% Computes selected residuals and raw threshold exceedance.
%
% State order:
% x = [u; v; w; phi; theta; psi; p; q; r; lon; lat; h]
%
% residual_selected order:
% 1 u residual
% 2 w residual
% 3 theta residual
% 4 q residual
% 5 altitude residual
% 6 phi residual
% 7 p residual
% 8 r residual
%--------------------------------------------------------------------------

%% Fixed-size outputs

residual_selected = zeros(8,1);
residual_norm     = 0.0;
exceeded_raw      = 0.0;

%% Compute selected residuals

residual_selected(1) = abs(x_meas_attacked(1)  - x_pred_unified(1));    % u
residual_selected(2) = abs(x_meas_attacked(3)  - x_pred_unified(3));    % w
residual_selected(3) = abs(x_meas_attacked(5)  - x_pred_unified(5));    % theta
residual_selected(4) = abs(x_meas_attacked(8)  - x_pred_unified(8));    % q
residual_selected(5) = abs(x_meas_attacked(12) - x_pred_unified(12));   % altitude
residual_selected(6) = abs(x_meas_attacked(4)  - x_pred_unified(4));    % phi
residual_selected(7) = abs(x_meas_attacked(7)  - x_pred_unified(7));    % p
residual_selected(8) = abs(x_meas_attacked(9)  - x_pred_unified(9));    % r

%% Residual norm

for i = 1:8
    residual_norm = residual_norm + residual_selected(i)^2;
end

residual_norm = sqrt(residual_norm);

%% Thresholds

u_threshold        = 5.0;          % m/s
w_threshold        = 2.0;          % m/s
theta_threshold    = 3*pi/180;     % rad
q_threshold        = 0.05;         % rad/s
altitude_threshold = 50.0;         % m
phi_threshold      = 5*pi/180;     % rad
p_threshold        = 0.05;         % rad/s
r_threshold        = 0.05;         % rad/s

%% Raw exceedance logic

if residual_selected(1) > u_threshold
    exceeded_raw = 1.0;
end

if residual_selected(2) > w_threshold
    exceeded_raw = 1.0;
end

if residual_selected(3) > theta_threshold
    exceeded_raw = 1.0;
end

if residual_selected(4) > q_threshold
    exceeded_raw = 1.0;
end

if residual_selected(5) > altitude_threshold
    exceeded_raw = 1.0;
end

if residual_selected(6) > phi_threshold
    exceeded_raw = 1.0;
end

if residual_selected(7) > p_threshold
    exceeded_raw = 1.0;
end

if residual_selected(8) > r_threshold
    exceeded_raw = 1.0;
end

end

== matlab function FYI_Twin_CyberResilient/Twin_States_Adapter/Geodetic Coordinates/LATITUDE ==
  data: VN input; phi_dot output; M input; h input
function phi_dot =Latitude_Rate(VN,M,h)
% Calculating the Rate of change of Latitude

phi_dot=VN/(M+h);
end

== matlab function FYI_Twin_CyberResilient/Twin_States_Adapter/Geodetic Coordinates/LONGITUDE ==
  data: VE input; gamma_dot output; N input; h input; phi input
function gamma_dot =Longitude_Rate(VE,N,h,phi)

% Calculating the Rate of change of the Longitude

gamma_dot=VE/((N+h)*cos(phi));
end
